simulink model "phaseplot"  (R2018b)
settings: Solver=ode8  StartTime=0.0  StopTime=10.0  FixedStep=0.001  RelTol=1e-3
libraries: simulink x1
settings Model: Creator=root  LastModifiedBy=root

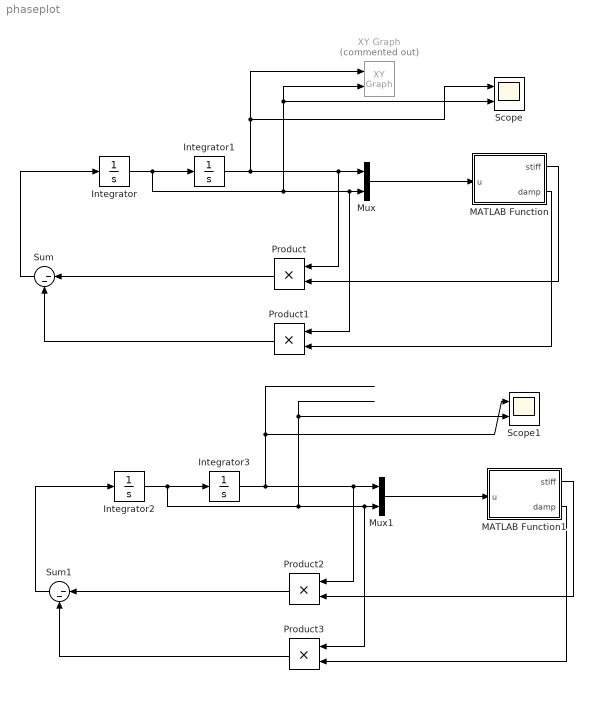
== system phaseplot ==
  Integrator : Integrator  InitialCondition=-1
  Integrator1 : Integrator  InitialCondition=1
  Integrator2 : Integrator  InitialCondition=-1
  Integrator3 : Integrator  InitialCondition=1
  MATLAB Function : MATLAB Function  TreatAsAtomicUnit=on
  MATLAB Function1 : MATLAB Function  TreatAsAtomicUnit=on
  Mux : Mux  Inputs=2
  Mux1 : Mux  Inputs=2
  Product{,1..3} (4 alike) : Product
  Scope : Scope  NumInputPorts=2
  Scope1 : Scope  NumInputPorts=2
  Sum : Sum  Inputs=|--
  Sum1 : Sum  Inputs=|--
  XY Graph : simulink/Sinks/XY Graph  Commented=on  xmin=-1  xmax=1  ymin=-1  ymax=1  st=-1
  wires:
  Integrator/1 -> Scope/2, XY Graph/2, Product1/1, Mux/2, Integrator1/1
  Mux/1 -> MATLAB Function/1(u)
  MATLAB Function/1(stiff) -> Product/2
  MATLAB Function/2(damp) -> Product1/2
  Product/1 -> Sum/1
  Product1/1 -> Sum/2
  Sum/1 -> Integrator/1
  Integrator1/1 -> Scope/1, XY Graph/1, Product/1, Mux/1
  Integrator3/1 -> Scope1/1, Product2/1, Mux1/1
  Mux1/1 -> MATLAB Function1/1(u)
  Integrator2/1 -> Scope1/2, Product3/1, Mux1/2, Integrator3/1
  Sum1/1 -> Integrator2/1
  MATLAB Function1/2(damp) -> Product3/2
  MATLAB Function1/1(stiff) -> Product2/2
  Product2/1 -> Sum1/1
  Product3/1 -> Sum1/2

== matlab function phaseplot/MATLAB Function1 ==
  data: u input; stiff output; damp output
function [stiff, damp] = fcn(u)
stiff_init = 4;
damp_init = 2 * sqrt(stiff_init);
rho_stiff = 1;
rho_damp = 1.5;
stiff = stiff_init * (1 + rho_stiff * (1 - u(1)));
damp = damp_init * (1 + rho_damp * (1 - u(1)));

== matlab function phaseplot/MATLAB Function ==
  data: u input; stiff output; damp output
function [stiff, damp] = fcn(u)
stiff = 4;
damp = 2 * sqrt(stiff);
